simulink model "Joystick20140103"  (R2012b)
settings: Solver=ode4  StartTime=0.0  StopTime=inf  FixedStep=sample_time  RelTol=1e-3
InitFcn:
  | sample_time=0.005;%0.004;%0.0025;%0.02;
  | sample_time_Vicon = 0.005;
  | DeltaT = 0.02;
  | g = 9.81;
  | H0 = g%0.3165;
  | Kl = 1;
  | 
  | Omega_r = 1.31;%for Horizontal reference
  | Zeta_r = 1; %for Horizontal reference
  | Omega = 1.31;%for Horizontal Control
  | Zeta = 0.7;    %for Horizontal Control
  | 
  | Omega_h_r = 2.2; %for vertical reference
  | Zeta_h_r = 1;  %for vertical reference
  | Omega_h = 2.2;    %for vertical control
  | Zeta_h = 1;         %for vertical control
  | PI=pi;
  | 
  | Mass = 1.1;
  | Acc_Max = 4;
  | Acc_Max_h = 4;
  | 
  | Max_RP = 60;
  | 
  | % for NN
  | n = 5;
  | r = 3;
  | n2 = 5;
  | NN_ST = 0.02;
  | 
  | GAMA_V = 3;
  | gama_V_e = 0.01;
  | 
  | GAMA_W = GAMA_V;
  | gama_W_e =0.01;
  | 
  | % deadzone
  | NN_Deadzone_Z = 0;
  | 
  | % inputs nomalizaton parameters
  | NN_Z_y_min = -3;
  | NN_Z_y_max = 0.5;
  | 
  | NN_Z_v_max = 8;
  | NN_Z_v_min = -NN_Z_v_max;
  | 
  | % alpha = 0.034;
  | alpha = 1;
  | % c_f = 0.0015;
  | c_f = 0.001;
  | c_y_tilt = 1*0.5;
  | 
  | %for WK paras
  | Heightcontrol = 0.08;
  | Scale_Factor=1;
  | yoffset=0;
  | 
  | load MaoBi_Oct04_2_int.mat
  | MB_Interp.time = [];
undefined symbols (not defined in the file or in its folder): DiscIntNeverNeededParam
libraries: simulink x12, X330_Control x4, vrlib x1
(part 2 of 2)

== system Joystick20140103/Vicon_Data/Raw Quad Pose from Vicon/Process Vicon Raw Data7/Flip_pi1/Flip_0_to_2pi/Flip_2pi ==
  Angle : Inport
  Bias : Bias  Bias=-2*pi
  Constant : Constant  Value=2*pi
  Data Type Duplicate : DataTypeDuplicate
  Modulo : Math  Operator=mod  SaturateOnIntegerOverflow=on
  Sign1 : Signum
  Switch : Switch
  Angle_Flip : Outport
  wires:
  Switch/1 -> Data Type Duplicate/2, Angle_Flip/1
  Bias/1 -> Switch/3
  Sign1/1 -> Switch/2
  Modulo/1 -> Switch/1, Bias/1
  Constant/1 -> Modulo/2
  Angle/1 -> Data Type Duplicate/1, Sign1/1, Modulo/1

== matlab function Joystick20140103/Joystick Mapping/check if quad are too close1 ==
  data: u input; ClawPWM output; counter data_store_memory; PWMclaw data_store_memory; JOYtrigger output; clawdone input double size=1
function [ClawPWM, JOYtrigger] = CLAW(u, clawdone)
global counter;
global PWMclaw;



if(clawdone==2)
    PWMclaw = 1200;
    ClawPWM = PWMclaw;
    JOYtrigger = u;
    
elseif(u~=1)
    if(PWMclaw==1690)
        counter = 1;
        ClawPWM = PWMclaw; 
        JOYtrigger = u;
    elseif (PWMclaw==1200)
        counter = 0;
        ClawPWM = PWMclaw;
        JOYtrigger = u;
    end
    

    
else
    if(counter==1)
        PWMclaw = 1200;
        ClawPWM = PWMclaw;
        JOYtrigger = u;
    elseif(counter==0)
        PWMclaw = 1690;
        ClawPWM = PWMclaw;
        JOYtrigger = u;
    end
    
end

ClawPWM = PWMclaw;
JOYtrigger = u;
   
end

== stateflow chart Joystick20140103/Planning/Trajectory Logic/UAV SF ==
  state AirBorne
    state Game
      state DecendPick
        state InZone
          state ResetJoyHoverAbove
            en:
            JoystickReset		= 1;
            PosDesired [0]		= 0;
            PosDesired [1]		= 0;
            PosDesired [2]		= -0.66;
            PWM 				= 1690;
          state Descent
            en:
            PosDesired [2] = -0.56;
          state CloseClaw1
            en:
            PWM = 1200;
            ClawDone =2;
          state Resumeback1
            en:
            ClawDone = 1;
          state Ascent1
            en:
            PosDesired [2]	 = -1;
          (default) -> ResetJoyHoverAbove
          ResetJoyHoverAbove -> Descent : [(abs(Pos[0]-PosDesired[0])+abs(Pos[1]-PosDesired[1]))<0.02]
          Descent -> CloseClaw1 : [abs(Pos[2]-PosDesired [2])<0.01]
          CloseClaw1 -> Ascent1 : after (1,sec)
          Ascent1 -> Resumeback1 : after (1.1,sec)
        state OutZone
          state ResetJoyDecent
            en:
            JoystickReset		= 1;
            PosDesired [2]		= -0.7;
            PWM 				= 1690;
          state CloseClaw
            en:
            PWM = 1200;
            ClawDone = 2;
          state Ascent
            en:
            PosDesired [2]		= -1;
          state Resumeback
            en:
            ClawDone = 1;
          (default) -> ResetJoyDecent : {PWM = 1690;}
          ResetJoyDecent -> CloseClaw : after (1.9,sec)
          CloseClaw -> Ascent : after (1.9,sec)
          Ascent -> Resumeback
        (default) -> (junction 1387)
        (junction 1387) -> OutZone [order 2] : [(TooClose[1]<=0.6)&&(TooClose[1]>=0.35)]
        (junction 1387) -> InZone [order 1] : [(TooClose[1]<0.35)]
      state JoystickCon
        du: PosDesired [0] = Joystick[0];
        PosDesired [1] = Joystick[1];
        PosDesired [2] = Joystick[2];
        PWM = Joystick[3];
      state ResetJoyStick1
        en:
        JoystickReset	= 0;
        ClawDone		= 0;
      state Flyaway
        en:
        XFly = TooClose[2];
        YFly = TooClose[3];
        Tooclosetrigger=1;
      state resetJoystick
        en:
        JoystickReset = 1;
        Tooclosetrigger=0;
      state Fly
        du:
        PosDesired[0] = (XFly-PosDesired[0])*1.7*DeltaT + PosDesired[0];
        PosDesired[1] = (YFly-PosDesired[1])*1.7*DeltaT + PosDesired[1];
      DecendPick -> ResetJoyStick1 : [ClawDone ==1]
      JoystickCon -> DecendPick [order 1] : [(TooClose[1]<=0.45)&&(JoystickTrigger==1)]
      (default) -> ResetJoyStick1
      ResetJoyStick1 -> JoystickCon
      resetJoystick -> ResetJoyStick1 [order 1] : [TooClose[0]==0]
      JoystickCon -> Flyaway [order 2] : [TooClose[0]==1]
      Flyaway -> Fly
      Fly -> resetJoystick : after (2.7,sec)
      resetJoystick -> Flyaway [order 2] : [TooClose[0]==1]
    state ResetJoyStick
      en:
      JoystickReset = 1;
      PosDesired [3] = 0;
    state TakeOff
      du:HoverThrottle = (H0 - HoverThrottle)*3*DeltaT + HoverThrottle ;
      PosDesired[2] = (-1.2- PosDesired[2])*1*DeltaT + PosDesired[2] ;
    state Safety
      state SafyHover
        du:PosDesired = Pos; PosDesired[2] = (-0.9-PosDesired[2])*2*DeltaT + PosDesired[2]; PWM = 1690;
      state OffloadPos
        du:
        PosDesired[0] = (0-PosDesired[0])*1*DeltaT + PosDesired[0];
        PosDesired[1] = (3.3-PosDesired[1])*1*DeltaT + PosDesired[1];
      state Descent2
        du:
        PosDesired[2] = (-0.57-PosDesired[2])*3*DeltaT + PosDesired[2];
      (default) -> SafyHover
      SafyHover -> OffloadPos : after (3, sec)
      OffloadPos -> Descent2 : after (4, sec)
    (default) -> TakeOff : {PosDesired = Pos;}
    TakeOff -> ResetJoyStick : after (7,sec)
    ResetJoyStick -> Game : [RC[5] > 0]
    Game -> Safety : [RC[5] < 0]
  note: Joystick[x]:
      |
      | 0. X-axis
      | 1. Y-axis
      | 2. Z-Axis
      | 3. PWM
      | 4. Trigger state
  state Landing
    state Descending
      en:PosDesired = Pos;
      du:PosDesired[2] = (0.2- PosDesired[2])*1*DeltaT + PosDesired[2] ;
    state CutThrottle
      en: PWM=1600;
      du:HoverThrottle = (0.0- HoverThrottle)*3*DeltaT + HoverThrottle ;
    (default) -> Descending
    Descending -> CutThrottle : [Pos[2] >(0.0 -0.2)]
  note: TooClose[x]:
      |
      | Where x=:
      | 0.	Bound
      | 1.	Q5 Current Radius
      | 2.	X
      | 3.	Y
  Landing -> AirBorne : [RC[6] > 0.5]
  AirBorne -> Landing : [RC[6] < -0.5]
  (default) -> Landing : {HoverThrottle = 0;}
  data: PosDesired output double size=4; HoverThrottle output double size=1; Mode output uint8 size=1; RC input size=8; Pos input size=4; PerchPos input size=4; DeltaT parameter size=1; H0 parameter size=1; Kl parameter size=1; VelCmd local double size=2 =0; PWM output double; PerchError input; PI parameter size=1; descentrate local double; Joystick input; TooClose input double; Tooclosetrigger local double =0; JoystickReset output double size=1; XFly local double size=1; YFly local double size=1; ClawDone output double size=1; JoystickTrigger input boolean size=1

== matlab function Joystick20140103/Planning/check if quad are too close ==
  data: Q1 input; Q2 input; Q3 input; Q4 input; Q5 input; BOUND output; Q5CR output; XJoy output [-3.5..3.5]; YJoy output [-3.5..3.5]; QD data_store_memory; PlatformAngle data_store_memory; XJoyOut data_store_memory; YJoyOut data_store_memory; XJoyIn data_store_memory; YJoyIn data_store_memory; TangentialAngle data_store_memory
function [BOUND, Q5CR,  XJoy, YJoy]   = Distance(Q1, Q2, Q3, Q4, Q5)

%  XJoyXInHalf, YJoyYInHalf, XTangentialInHalf, YTangentialInHalf,  XTangentialOutHalf, YTangentialOutHalf, XJoyXOutHalf, YJoyYOutHalf

global QD;
global PlatformAngle;
global XJoyIn;
global YJoyIn;
global XJoyOut;
global YJoyOut;
global TangentialAngle;

%Distance between Joystick Quad and Formation Quad.
DQ1 = sqrt((Q5(1)-Q1(1))^2 + (Q5(2)-Q1(2))^2);
DQ2 = sqrt((Q5(1)-Q2(1))^2 + (Q5(2)-Q2(2))^2);
DQ3 = sqrt((Q5(1)-Q3(1))^2 + (Q5(2)-Q3(2))^2);
DQ4 = sqrt((Q5(1)-Q4(1))^2 + (Q5(2)-Q4(2))^2);

%Joystick quad current distance away from platform.


% PlatformAngle = atan2((Q5(2)-Platform(2)),(Q5(1)-Platform(1)));
PlatformAngle = atan2((Q5(1)),(Q5(2)));

%Coordinates to fly outwards while remaining 3m radius away from platform.

XJoyOut     = 3.4*sin(PlatformAngle);
YJoyOut     = 3.4*cos(PlatformAngle);

XJoyIn      = 0.5*sin(PlatformAngle);
YJoyIn      = 0.5*cos(PlatformAngle);

    
if ((DQ1<1.13)||(DQ2<1.13)||(DQ3<1.13)||(DQ4<1.13))
    QD          = 1;
    BOUND       = QD;
    Q5CR        = sqrt(Q5(1)^2 + Q5(2)^2);
      
   if(Q5CR<1.75)
        XJoy    = XJoyIn;
        YJoy    = YJoyIn;
   
   elseif ((Q5CR>=1.75)&&(Q5CR<=2.3))    
        TangentialAngle = acos((sqrt(Q5(1)^2 + Q5(2)^2))/3.3);
        XJoy    = YJoyOut*sin(TangentialAngle) + XJoyOut*cos(TangentialAngle);
        YJoy    = YJoyOut*cos(TangentialAngle) - XJoyOut*sin(TangentialAngle);  
   
   
   else
        XJoy    = XJoyOut;
        YJoy    = YJoyOut;
       
    end
    
       

else
    QD          = 0;
    BOUND       = QD;
    Q5CR        = sqrt(Q5(1)^2 + Q5(2)^2);
    
    if(Q5CR<2)
        XJoy    = XJoyIn;
        YJoy    = YJoyIn;
     
   
   else
        XJoy    = XJoyOut;
        YJoy    = YJoyOut;       
    
        
    end

end
end
